simulink model "Modelo_R2023b"  (R2023b)
settings: Solver=VariableStepAuto  StartTime=0.0  StopTime=10.0  RelTol=1e-3
model workspace (MAT data in the model file):
  DC_Joint_J = 0.192319441127
  DC_Motor_D = 0.4
  DC_Motor_H = 0.192915716702
  DC_Motor_I = 1
  DC_Motor_J = 0.2131632295
  DC_Motor_Lower_Sat_Ref = -18
  DC_Motor_NLC = 0.11
  DC_Motor_NLS = 10000
  DC_Motor_P = 0.20625
  DC_Motor_ST = 0.0494309
  DC_Motor_TG = 0.95
  DC_Motor_Upper_Sat_Ref = 18
  DC_Motor_V = 12
  DRV_Deadzone_U = 128
  DRV_Motor_BTH = 0.001
  DRV_Motor_ETH = 0.15625
  DRV_Motor_FDR = 0.195188957589
  DRV_Motor_RTH = 0.001
  DRV_Motor_TBR = 0.10371374274
  MOTOR_Period_T = 0.01
  MOTOR_WHEEL_LPF : object (value not decoded)
  Robot_L = 0.15
  Robot_W = 0.15
  Robot_init_th = 0
  Robot_init_x = 0
  Robot_init_y = 0
  Robot_mm_to_m = 0.001
  Robot_wheel_radius = 0.05
  Robot_wheel_x_offset = 150
  Robot_wheel_y_offset = 102.5
  Robot_wheel_z_offset = 2
  Roller_Contact_df = 0.3
  Roller_Contact_dm = 1000
  Roller_Contact_sf = 0.5
  Roller_Contact_st = 1000000
  Roller_Joint_Friction = 0
  SIM_Base_Period_T = 0.001
  SIM_CTRL_Period_T = 0.1
  SIM_Floor_Height = 8.7
  SIM_Floor_Thick = 0.2
  SIM_Floor_Width = 9
  Sig : Simulink.Signal (value not decoded)
  Traj_ref = [0 0.1 0.2 0.3 0.4 0.5 0.6 0.7 0.8 0.9 1 0 ... (22 elements, 11x2)]
undefined symbols (not defined in the file): DiscIntNeverNeededParam, X, Y, Z
libraries: sm_lib x185, nesl_utility x37, fl_lib x32, ee_lib x12, simulink x8, aerolibconvert2 x4, cstblocks x4, sharedtransform x1, dspsigops x1
(part 4 of 4)

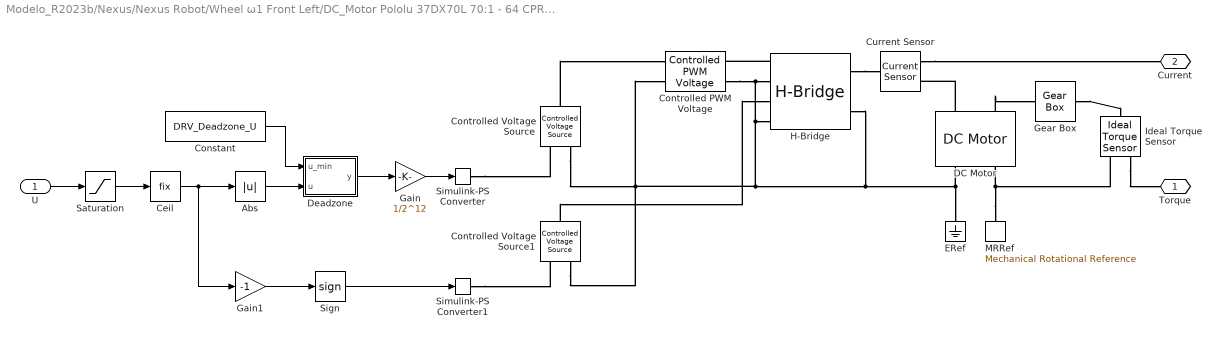
== system Modelo_R2023b/Nexus/Nexus Robot/Wheel ω1 Front Left/DC_Motor Pololu 37DX70L 70:1 - 64 CPR/Electrical ==
  U : Inport
  Abs : Abs  SaturateOnIntegerOverflow=off
  Ceil : Rounding  Operator=fix
  Constant : Constant  Value=DRV_Deadzone_U
  Controlled PWM Voltage : ee_lib/Integrated Circuits/Controlled PWM Voltage  F=1526 Hz  TD=0 s  pulse_width_offset=0 s  pulse_min=0 s  pwm_or_av=2  event_type=1  sample_time=5e-6 s  Vmin=0 V  Vmax=1 V  Vm=5 V  u_min=0  u_max=1
  Controlled Voltage Source : fl_lib/Electrical/Electrical Sources/Controlled Voltage Source
  Controlled Voltage Source1 : fl_lib/Electrical/Electrical Sources/Controlled Voltage Source
  Current Sensor : fl_lib/Electrical/Electrical Sensors/Current Sensor
  DC Motor : ee_lib/Electromechanical/Brushed Motors/DC Motor  field_option=ee.enum.field_option.pm  Rf=100 Ohm  Lf=1 H  Laf=0.15 H  If0=0 A  parameterization=ee.enum.dcparam_option.torque_speed  Ra=DC_Motor_R Ohm  La=DC_Motor_H H  emf_or_torque=ee.enum.emf_or_torque.kv  Kv=DC_Motor_K V/(rad/s)  Ki=6.876e-04 N*m/A  T_stall=DC_Motor_ST N*m  w_max=DC_Motor_NLS rpm  w_rated=150 rpm  P_rated=10 W  V_rated=nomV V  lam_param=ee.enum.lam_param.current  i_noload=0.11 A  V_i_noload=nomV V  J=DC_Motor_J kg*m^2  lam=DC_Motor_D N*m/(rad/s)  speed0=0 rpm  enable_fault_armature=simscape.enum.onoff.off  rev_faulted=1 / 3  G_faulted_armature=1e-5 S  fault_trigger_armature=ee.enum.faults.faultTrigger.temporal  t_fault_armature=1 s  max_permissible_current_armature=inf A  t_fail_on_current_armature=1 s  enable_fault_field=simscape.enum.onoff.off  G_faulted_field=1e-5 S  fault_trigger_field=ee.enum.faults.faultTrigger.temporal  t_fault_field=1 s  max_permissible_current_field=inf A  t_fail_on_current_field=1 s  fault_action=simscape.enum.assert.action.none  alpha=3.93e-3 1/K  Tmeas=25 degC  thermal_mass=100 J/K  initial_temperature=25 degC
  Deadzone : MATLAB Function  TreatAsAtomicUnit=on
  ERef : fl_lib/Electrical/Electrical Elements/Electrical Reference
  Gain : Gain  Gain=1/2^12
  Gain1 : Gain  Gain=-1
  Gear Box : fl_lib/Mechanical/Mechanisms/Gear Box  ratio=70  t_in_specify=off  t_in_priority=None  t_in=0 N*m  t_in_nominal_specify=off  t_in_nominal_unit=N*m  t_in_nominal_value=1  t_out_specify=off  t_out_priority=None  t_out=0 N*m  t_out_nominal_specify=off  t_out_nominal_unit=N*m  t_out_nominal_value=1
  H-Bridge : ee_lib/Semiconductors & Converters/Converters/H-Bridge  supply_ports=ee.enum.supply_ports.hidesupply  pwm_or_av=ee.enum.pwm_or_av.averaged  regenerative_braking_mode=ee.enum.converters.regenerative_braking_mode.always_enabled  discontinuous=ee.enum.current_profile.continuous  freewheeling_mode=ee.enum.converters.freewheeling_mode.one_switch_one_diode  Rload=3.38+0.1 Ohm  Lload=1e-5 H  F=4 kHz  Venable=DRV_Motor_ETH V  Vmax=5 V  Vreverse=DRV_Motor_RTH V  Vbrake=DRV_Motor_BTH V  Vm=nomV V  Ron=DRV_Motor_TBR Ohm  Don=DRV_Motor_FDR Ohm  Goff=1e-6 S  Tmeas=298.15 K  Ron2=0.1 Ohm  Don2=0.05 Ohm  Tmeas2=398.15 K  thermal_mass=100 J/K  initial_temperature=298.15 K
  Ideal Torque Sensor : fl_lib/Mechanical/Mechanical Sensors/Ideal Torque Sensor
  MRRef : fl_lib/Mechanical/Rotational Elements/Mechanical Rotational Reference
  Saturation : Saturate  UpperLimit=4096  LowerLimit=-4096
  Sign : Signum
  Simulink-PS Converter : nesl_utility/Simulink-PS Converter  PhysicalDomain=network_engine_domain  SubClassName=ps_input  LeftPortType=input  RightPortType=output  PseudoPeriodic=off  Frequencies=[]  NoiseDistribution=none  NoiseParameters=[]  Unit=V  AffineConversion=off  FilteringAndDerivatives=provide  SimscapeFilterOrder=1  InputFilterTimeConstant=0.001  UdotUserProvided=0
  Simulink-PS Converter1 : nesl_utility/Simulink-PS Converter  PhysicalDomain=network_engine_domain  SubClassName=ps_input  LeftPortType=input  RightPortType=output  PseudoPeriodic=off  Frequencies=[]  NoiseDistribution=none  NoiseParameters=[]  Unit=V  AffineConversion=off  FilteringAndDerivatives=provide  SimscapeFilterOrder=1  InputFilterTimeConstant=0.001  UdotUserProvided=0
  Torque : PMIOPort  Side=Right
  Current : PMIOPort  Port=2  Side=Right
  wires:
  Saturation/1 -> Ceil/1
  Sign/1 -> Simulink-PS Converter1/1
  Gain/1 -> Simulink-PS Converter/1
  U/1 -> Saturation/1
  Abs/1 -> Deadzone/2(u)
  Ceil/1 -> Gain1/1, Abs/1
  Deadzone/1(y) -> Gain/1
  Gain1/1 -> Sign/1
  Constant/1 -> Deadzone/1(u_min)
  connections:
  H-Bridge/RConn2 -- DC Motor/RConn1 -- ERef/LConn1 -- Controlled Voltage Source1/RConn2 -- Controlled Voltage Source/RConn2 -- Controlled PWM Voltage/LConn2 -- H-Bridge/LConn4 -- H-Bridge/LConn2 -- Controlled PWM Voltage/RConn2
  MRRef/LConn1 -- Ideal Torque Sensor/RConn1 -- DC Motor/RConn2
  H-Bridge/RConn1 -- Current Sensor/LConn1
  DC Motor/LConn1 -- Current Sensor/RConn2
  H-Bridge/LConn1 -- Controlled PWM Voltage/RConn1
  Current Sensor/RConn1 -- Current/RConn1
  Controlled Voltage Source/LConn1 -- Controlled PWM Voltage/LConn1
  Simulink-PS Converter/RConn1 -- Controlled Voltage Source/RConn1
  Ideal Torque Sensor/RConn2 -- Torque/RConn1
  DC Motor/LConn2 -- Gear Box/LConn1
  Gear Box/RConn1 -- Ideal Torque Sensor/LConn1
  Simulink-PS Converter1/RConn1 -- Controlled Voltage Source1/RConn1
  Controlled Voltage Source1/LConn1 -- H-Bridge/LConn3

== system Modelo_R2023b/Nexus/Nexus Robot/Wheel ω1 Front Left/DC_Motor Pololu 37DX70L 70:1 - 64 CPR/Mechanics ==
  Axis : sm_lib/Body Elements/File Solid  ExtGeomFileName=c_MG37D_Eje.stp  UnitType=FromFile  ExtGeomFileUnits=m  StepReaderType=HEX  ExportConvexHullGeometry=off  InertiaType=CalculateFromGeometry  Mass=1  MassUnits=kg  CenterOfMass=[0 0 0]  CenterOfMassUnits=m  MomentsOfInertia=[1 1 1]  MomentsOfInertiaUnits=kg*m^2  ProductsOfInertia=[0 0 0]  ProductsOfInertiaUnits=kg*m^2  BasedOnType=Density  Density=7850  DensityUnits=kg/m^3  DoExposeReferenceFrame=on  SerializedFrames=<Frames><Frame><Id>Frame1</Id><Value><Name>F1</Name><Origin><Source>GeometricFeature</Source><FeatureName>circular curve 6</FeatureName></Origin><PrimaryAxis><DefinedDirection>+Z</DefinedDirection><Source>ReferenceFrame</Source><SourceDirection>+Z</SourceDirection><FeatureName></FeatureName></PrimaryAxis><SecondaryAxis><DefinedDirection>+X</DefinedDirection><Source>ReferenceFrame</Source><SourceDirection>+X</SourceDirection><FeatureName></FeatureName></SecondaryAxis></Value></Frame></Frames>  GraphicType=FromGeometry  MarkerShape=Sphere  MarkerSize=10  GraphicVisPropType=SimpleVisualProperties  GraphicDiffuseColor=[0.8 0.8 0.8]  GraphicSpecularColor=[0.5 0.5 0.5 1.0]  GraphicAmbientColor=[0.15 0.15 0.15 1.0]  GraphicEmissiveColor=[0.0 0.0 0.0 1.0]  GraphicShininess=75  GraphicOpacity=1.0
  PS Gain : fl_lib/Physical Signals/Functions/PS Gain  gain=DC_Motor_TG
  Revolute Joint : sm_lib/Joints/Revolute Joint  JointMode=Normal  SenseConstraintForce=off  SenseConstraintForceX=off  SenseConstraintForceY=off  SenseConstraintForceZ=off  SenseConstraintTorque=off  SenseConstraintTorqueX=off  SenseConstraintTorqueY=off  SenseConstraintTorqueZ=off  SenseTotalForce=off  SenseTotalForceX=off  SenseTotalForceY=off  SenseTotalForceZ=off  SenseTotalTorque=off  SenseTotalTorqueX=off  SenseTotalTorqueY=off  SenseTotalTorqueZ=off  CompositeWrenchDir=FollowerOnBase  CompositeWrenchFrame=BaseFrame  EquilibriumPosition=0  EquilibriumPositionUnits=deg  SpringStiffness=0  SpringStiffnessUnits=N*m/deg  DampingCoefficient=DC_Joint_J  DampingCoefficientUnits=N*m/(rad/s)  TorqueActuationMode=InputTorque  MotionActuationMode=ComputedMotion  SensePosition=on  SenseVelocity=on  SenseAcceleration=off  SenseTorqueForce=off  SenseLowerLimitTorqueForce=off  SenseUpperLimitTorqueForce=off  LowerLimitSpecify=off  LowerLimitBound=-90  LowerLimitBoundUnits=deg  LowerLimitStiffness=1e4  LowerLimitStiffnessUnits=N*m/deg  LowerLimitDamping=10  LowerLimitDampingUnits=N*m/(deg/s)  LowerLimitTransitionRegionWidth=0.1  LowerLimitTransitionRegionWidthUnits=deg  UpperLimitSpecify=off  UpperLimitBound=90  UpperLimitBoundUnits=deg  UpperLimitStiffness=1e4  UpperLimitStiffnessUnits=N*m/deg  UpperLimitDamping=10  UpperLimitDampingUnits=N*m/(deg/s)  UpperLimitTransitionRegionWidth=0.1  UpperLimitTransitionRegionWidthUnits=deg  PositionTargetSpecify=off  PositionTargetPriority=High  PositionTargetValue=0  PositionTargetValueUnits=deg  VelocityTargetSpecify=off  VelocityTargetPriority=High  VelocityTargetValue=0  VelocityTargetValueUnits=deg/s
  FW : PMIOPort  Side=Left
  τ : PMIOPort  Port=2  Side=Left
  Wheel : PMIOPort  Port=3  Side=Right
  θ : PMIOPort  Port=4  Side=Right
  ω : PMIOPort  Port=5  Side=Right
  connections:
  Revolute Joint/RConn2 -- θ/RConn1
  FW/RConn1 -- Revolute Joint/LConn1
  Axis/RConn1 -- Revolute Joint/RConn1
  PS Gain/LConn1 -- τ/RConn1
  Revolute Joint/RConn3 -- ω/RConn1
  Revolute Joint/LConn2 -- PS Gain/RConn1
  Wheel/RConn1 -- Axis/LConn1

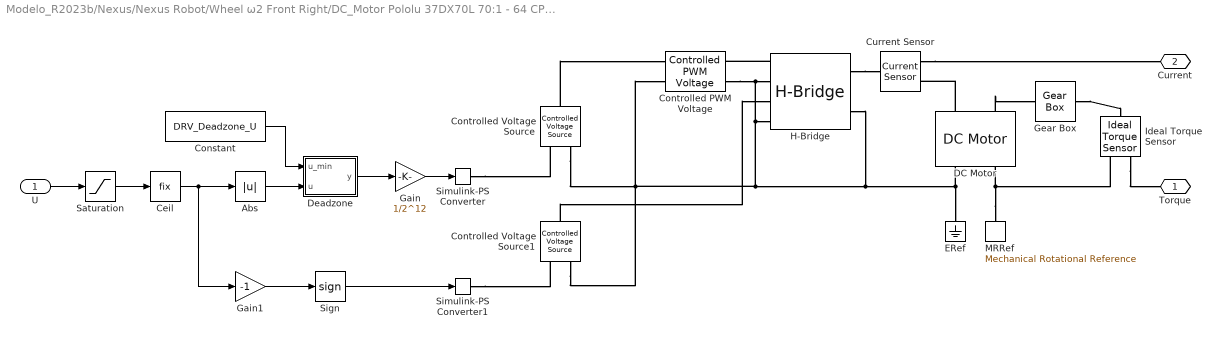
== system Modelo_R2023b/Nexus/Nexus Robot/Wheel ω2 Front Right/DC_Motor Pololu 37DX70L 70:1 - 64 CPR/Electrical ==
  U : Inport
  Abs : Abs  SaturateOnIntegerOverflow=off
  Ceil : Rounding  Operator=fix
  Constant : Constant  Value=DRV_Deadzone_U
  Controlled PWM Voltage : ee_lib/Integrated Circuits/Controlled PWM Voltage  F=1526 Hz  TD=0 s  pulse_width_offset=0 s  pulse_min=0 s  pwm_or_av=2  event_type=1  sample_time=5e-6 s  Vmin=0 V  Vmax=1 V  Vm=5 V  u_min=0  u_max=1
  Controlled Voltage Source : fl_lib/Electrical/Electrical Sources/Controlled Voltage Source
  Controlled Voltage Source1 : fl_lib/Electrical/Electrical Sources/Controlled Voltage Source
  Current Sensor : fl_lib/Electrical/Electrical Sensors/Current Sensor
  DC Motor : ee_lib/Electromechanical/Brushed Motors/DC Motor  field_option=ee.enum.field_option.pm  Rf=100 Ohm  Lf=1 H  Laf=0.15 H  If0=0 A  parameterization=ee.enum.dcparam_option.torque_speed  Ra=DC_Motor_R Ohm  La=DC_Motor_H H  emf_or_torque=ee.enum.emf_or_torque.kv  Kv=DC_Motor_K V/(rad/s)  Ki=6.876e-04 N*m/A  T_stall=DC_Motor_ST N*m  w_max=DC_Motor_NLS rpm  w_rated=150 rpm  P_rated=10 W  V_rated=nomV V  lam_param=ee.enum.lam_param.current  i_noload=0.11 A  V_i_noload=nomV V  J=DC_Motor_J kg*m^2  lam=DC_Motor_D N*m/(rad/s)  speed0=0 rpm  enable_fault_armature=simscape.enum.onoff.off  rev_faulted=1 / 3  G_faulted_armature=1e-5 S  fault_trigger_armature=ee.enum.faults.faultTrigger.temporal  t_fault_armature=1 s  max_permissible_current_armature=inf A  t_fail_on_current_armature=1 s  enable_fault_field=simscape.enum.onoff.off  G_faulted_field=1e-5 S  fault_trigger_field=ee.enum.faults.faultTrigger.temporal  t_fault_field=1 s  max_permissible_current_field=inf A  t_fail_on_current_field=1 s  fault_action=simscape.enum.assert.action.none  alpha=3.93e-3 1/K  Tmeas=25 degC  thermal_mass=100 J/K  initial_temperature=25 degC
  Deadzone : MATLAB Function  TreatAsAtomicUnit=on
  ERef : fl_lib/Electrical/Electrical Elements/Electrical Reference
  Gain : Gain  Gain=1/2^12
  Gain1 : Gain  Gain=-1
  Gear Box : fl_lib/Mechanical/Mechanisms/Gear Box  ratio=70  t_in_specify=off  t_in_priority=None  t_in=0 N*m  t_in_nominal_specify=off  t_in_nominal_unit=N*m  t_in_nominal_value=1  t_out_specify=off  t_out_priority=None  t_out=0 N*m  t_out_nominal_specify=off  t_out_nominal_unit=N*m  t_out_nominal_value=1
  H-Bridge : ee_lib/Semiconductors & Converters/Converters/H-Bridge  supply_ports=ee.enum.supply_ports.hidesupply  pwm_or_av=ee.enum.pwm_or_av.averaged  regenerative_braking_mode=ee.enum.converters.regenerative_braking_mode.always_enabled  discontinuous=ee.enum.current_profile.continuous  freewheeling_mode=ee.enum.converters.freewheeling_mode.one_switch_one_diode  Rload=3.38+0.1 Ohm  Lload=1e-5 H  F=4 kHz  Venable=DRV_Motor_ETH V  Vmax=5 V  Vreverse=DRV_Motor_RTH V  Vbrake=DRV_Motor_BTH V  Vm=nomV V  Ron=DRV_Motor_TBR Ohm  Don=DRV_Motor_FDR Ohm  Goff=1e-6 S  Tmeas=298.15 K  Ron2=0.1 Ohm  Don2=0.05 Ohm  Tmeas2=398.15 K  thermal_mass=100 J/K  initial_temperature=298.15 K
  Ideal Torque Sensor : fl_lib/Mechanical/Mechanical Sensors/Ideal Torque Sensor
  MRRef : fl_lib/Mechanical/Rotational Elements/Mechanical Rotational Reference
  Saturation : Saturate  UpperLimit=4096  LowerLimit=-4096
  Sign : Signum
  Simulink-PS Converter : nesl_utility/Simulink-PS Converter  PhysicalDomain=network_engine_domain  SubClassName=ps_input  LeftPortType=input  RightPortType=output  PseudoPeriodic=off  Frequencies=[]  NoiseDistribution=none  NoiseParameters=[]  Unit=V  AffineConversion=off  FilteringAndDerivatives=provide  SimscapeFilterOrder=1  InputFilterTimeConstant=0.001  UdotUserProvided=0
  Simulink-PS Converter1 : nesl_utility/Simulink-PS Converter  PhysicalDomain=network_engine_domain  SubClassName=ps_input  LeftPortType=input  RightPortType=output  PseudoPeriodic=off  Frequencies=[]  NoiseDistribution=none  NoiseParameters=[]  Unit=V  AffineConversion=off  FilteringAndDerivatives=provide  SimscapeFilterOrder=1  InputFilterTimeConstant=0.001  UdotUserProvided=0
  Torque : PMIOPort  Side=Right
  Current : PMIOPort  Port=2  Side=Right
  wires:
  Saturation/1 -> Ceil/1
  Sign/1 -> Simulink-PS Converter1/1
  Gain/1 -> Simulink-PS Converter/1
  U/1 -> Saturation/1
  Abs/1 -> Deadzone/2(u)
  Ceil/1 -> Gain1/1, Abs/1
  Deadzone/1(y) -> Gain/1
  Gain1/1 -> Sign/1
  Constant/1 -> Deadzone/1(u_min)
  connections:
  H-Bridge/RConn2 -- DC Motor/RConn1 -- ERef/LConn1 -- Controlled Voltage Source1/RConn2 -- Controlled Voltage Source/RConn2 -- Controlled PWM Voltage/LConn2 -- H-Bridge/LConn4 -- H-Bridge/LConn2 -- Controlled PWM Voltage/RConn2
  MRRef/LConn1 -- Ideal Torque Sensor/RConn1 -- DC Motor/RConn2
  H-Bridge/RConn1 -- Current Sensor/LConn1
  DC Motor/LConn1 -- Current Sensor/RConn2
  H-Bridge/LConn1 -- Controlled PWM Voltage/RConn1
  Current Sensor/RConn1 -- Current/RConn1
  Controlled Voltage Source/LConn1 -- Controlled PWM Voltage/LConn1
  Simulink-PS Converter/RConn1 -- Controlled Voltage Source/RConn1
  Ideal Torque Sensor/RConn2 -- Torque/RConn1
  DC Motor/LConn2 -- Gear Box/LConn1
  Gear Box/RConn1 -- Ideal Torque Sensor/LConn1
  Simulink-PS Converter1/RConn1 -- Controlled Voltage Source1/RConn1
  Controlled Voltage Source1/LConn1 -- H-Bridge/LConn3

== system Modelo_R2023b/Nexus/Nexus Robot/Wheel ω2 Front Right/DC_Motor Pololu 37DX70L 70:1 - 64 CPR/Mechanics ==
  Axis : sm_lib/Body Elements/File Solid  ExtGeomFileName=c_MG37D_Eje.stp  UnitType=FromFile  ExtGeomFileUnits=m  StepReaderType=HEX  ExportConvexHullGeometry=off  InertiaType=CalculateFromGeometry  Mass=1  MassUnits=kg  CenterOfMass=[0 0 0]  CenterOfMassUnits=m  MomentsOfInertia=[1 1 1]  MomentsOfInertiaUnits=kg*m^2  ProductsOfInertia=[0 0 0]  ProductsOfInertiaUnits=kg*m^2  BasedOnType=Density  Density=7850  DensityUnits=kg/m^3  DoExposeReferenceFrame=on  SerializedFrames=<Frames><Frame><Id>Frame1</Id><Value><Name>F1</Name><Origin><Source>GeometricFeature</Source><FeatureName>circular curve 6</FeatureName></Origin><PrimaryAxis><DefinedDirection>+Z</DefinedDirection><Source>ReferenceFrame</Source><SourceDirection>+Z</SourceDirection><FeatureName></FeatureName></PrimaryAxis><SecondaryAxis><DefinedDirection>+X</DefinedDirection><Source>ReferenceFrame</Source><SourceDirection>+X</SourceDirection><FeatureName></FeatureName></SecondaryAxis></Value></Frame></Frames>  GraphicType=FromGeometry  MarkerShape=Sphere  MarkerSize=10  GraphicVisPropType=SimpleVisualProperties  GraphicDiffuseColor=[0.8 0.8 0.8]  GraphicSpecularColor=[0.5 0.5 0.5 1.0]  GraphicAmbientColor=[0.15 0.15 0.15 1.0]  GraphicEmissiveColor=[0.0 0.0 0.0 1.0]  GraphicShininess=75  GraphicOpacity=1.0
  PS Gain : fl_lib/Physical Signals/Functions/PS Gain  gain=DC_Motor_TG
  Revolute Joint : sm_lib/Joints/Revolute Joint  JointMode=Normal  SenseConstraintForce=off  SenseConstraintForceX=off  SenseConstraintForceY=off  SenseConstraintForceZ=off  SenseConstraintTorque=off  SenseConstraintTorqueX=off  SenseConstraintTorqueY=off  SenseConstraintTorqueZ=off  SenseTotalForce=off  SenseTotalForceX=off  SenseTotalForceY=off  SenseTotalForceZ=off  SenseTotalTorque=off  SenseTotalTorqueX=off  SenseTotalTorqueY=off  SenseTotalTorqueZ=off  CompositeWrenchDir=FollowerOnBase  CompositeWrenchFrame=BaseFrame  EquilibriumPosition=0  EquilibriumPositionUnits=deg  SpringStiffness=0  SpringStiffnessUnits=N*m/deg  DampingCoefficient=DC_Joint_J  DampingCoefficientUnits=N*m/(rad/s)  TorqueActuationMode=InputTorque  MotionActuationMode=ComputedMotion  SensePosition=on  SenseVelocity=on  SenseAcceleration=off  SenseTorqueForce=off  SenseLowerLimitTorqueForce=off  SenseUpperLimitTorqueForce=off  LowerLimitSpecify=off  LowerLimitBound=-90  LowerLimitBoundUnits=deg  LowerLimitStiffness=1e4  LowerLimitStiffnessUnits=N*m/deg  LowerLimitDamping=10  LowerLimitDampingUnits=N*m/(deg/s)  LowerLimitTransitionRegionWidth=0.1  LowerLimitTransitionRegionWidthUnits=deg  UpperLimitSpecify=off  UpperLimitBound=90  UpperLimitBoundUnits=deg  UpperLimitStiffness=1e4  UpperLimitStiffnessUnits=N*m/deg  UpperLimitDamping=10  UpperLimitDampingUnits=N*m/(deg/s)  UpperLimitTransitionRegionWidth=0.1  UpperLimitTransitionRegionWidthUnits=deg  PositionTargetSpecify=off  PositionTargetPriority=High  PositionTargetValue=0  PositionTargetValueUnits=deg  VelocityTargetSpecify=off  VelocityTargetPriority=High  VelocityTargetValue=0  VelocityTargetValueUnits=deg/s
  FW : PMIOPort  Side=Left
  τ : PMIOPort  Port=2  Side=Left
  Wheel : PMIOPort  Port=3  Side=Right
  θ : PMIOPort  Port=4  Side=Right
  ω : PMIOPort  Port=5  Side=Right
  connections:
  Revolute Joint/RConn2 -- θ/RConn1
  FW/RConn1 -- Revolute Joint/LConn1
  Axis/RConn1 -- Revolute Joint/RConn1
  PS Gain/LConn1 -- τ/RConn1
  Revolute Joint/RConn3 -- ω/RConn1
  Revolute Joint/LConn2 -- PS Gain/RConn1
  Wheel/RConn1 -- Axis/LConn1

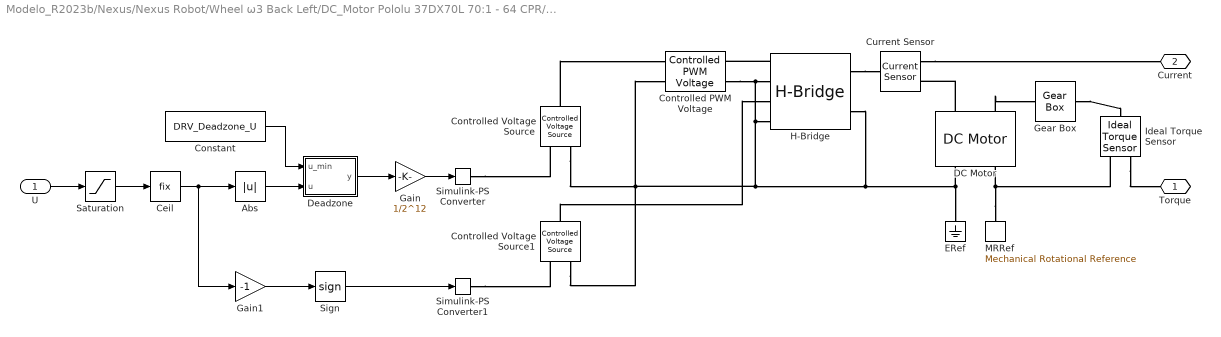
== system Modelo_R2023b/Nexus/Nexus Robot/Wheel ω3 Back Left/DC_Motor Pololu 37DX70L 70:1 - 64 CPR/Electrical ==
  U : Inport
  Abs : Abs  SaturateOnIntegerOverflow=off
  Ceil : Rounding  Operator=fix
  Constant : Constant  Value=DRV_Deadzone_U
  Controlled PWM Voltage : ee_lib/Integrated Circuits/Controlled PWM Voltage  F=1526 Hz  TD=0 s  pulse_width_offset=0 s  pulse_min=0 s  pwm_or_av=2  event_type=1  sample_time=5e-6 s  Vmin=0 V  Vmax=1 V  Vm=5 V  u_min=0  u_max=1
  Controlled Voltage Source : fl_lib/Electrical/Electrical Sources/Controlled Voltage Source
  Controlled Voltage Source1 : fl_lib/Electrical/Electrical Sources/Controlled Voltage Source
  Current Sensor : fl_lib/Electrical/Electrical Sensors/Current Sensor
  DC Motor : ee_lib/Electromechanical/Brushed Motors/DC Motor  field_option=ee.enum.field_option.pm  Rf=100 Ohm  Lf=1 H  Laf=0.15 H  If0=0 A  parameterization=ee.enum.dcparam_option.torque_speed  Ra=DC_Motor_R Ohm  La=DC_Motor_H H  emf_or_torque=ee.enum.emf_or_torque.kv  Kv=DC_Motor_K V/(rad/s)  Ki=6.876e-04 N*m/A  T_stall=DC_Motor_ST N*m  w_max=DC_Motor_NLS rpm  w_rated=150 rpm  P_rated=10 W  V_rated=nomV V  lam_param=ee.enum.lam_param.current  i_noload=0.11 A  V_i_noload=nomV V  J=DC_Motor_J kg*m^2  lam=DC_Motor_D N*m/(rad/s)  speed0=0 rpm  enable_fault_armature=simscape.enum.onoff.off  rev_faulted=1 / 3  G_faulted_armature=1e-5 S  fault_trigger_armature=ee.enum.faults.faultTrigger.temporal  t_fault_armature=1 s  max_permissible_current_armature=inf A  t_fail_on_current_armature=1 s  enable_fault_field=simscape.enum.onoff.off  G_faulted_field=1e-5 S  fault_trigger_field=ee.enum.faults.faultTrigger.temporal  t_fault_field=1 s  max_permissible_current_field=inf A  t_fail_on_current_field=1 s  fault_action=simscape.enum.assert.action.none  alpha=3.93e-3 1/K  Tmeas=25 degC  thermal_mass=100 J/K  initial_temperature=25 degC
  Deadzone : MATLAB Function  TreatAsAtomicUnit=on
  ERef : fl_lib/Electrical/Electrical Elements/Electrical Reference
  Gain : Gain  Gain=1/2^12
  Gain1 : Gain  Gain=-1
  Gear Box : fl_lib/Mechanical/Mechanisms/Gear Box  ratio=70  t_in_specify=off  t_in_priority=None  t_in=0 N*m  t_in_nominal_specify=off  t_in_nominal_unit=N*m  t_in_nominal_value=1  t_out_specify=off  t_out_priority=None  t_out=0 N*m  t_out_nominal_specify=off  t_out_nominal_unit=N*m  t_out_nominal_value=1
  H-Bridge : ee_lib/Semiconductors & Converters/Converters/H-Bridge  supply_ports=ee.enum.supply_ports.hidesupply  pwm_or_av=ee.enum.pwm_or_av.averaged  regenerative_braking_mode=ee.enum.converters.regenerative_braking_mode.always_enabled  discontinuous=ee.enum.current_profile.continuous  freewheeling_mode=ee.enum.converters.freewheeling_mode.one_switch_one_diode  Rload=3.38+0.1 Ohm  Lload=1e-5 H  F=4 kHz  Venable=DRV_Motor_ETH V  Vmax=5 V  Vreverse=DRV_Motor_RTH V  Vbrake=DRV_Motor_BTH V  Vm=nomV V  Ron=DRV_Motor_TBR Ohm  Don=DRV_Motor_FDR Ohm  Goff=1e-6 S  Tmeas=298.15 K  Ron2=0.1 Ohm  Don2=0.05 Ohm  Tmeas2=398.15 K  thermal_mass=100 J/K  initial_temperature=298.15 K
  Ideal Torque Sensor : fl_lib/Mechanical/Mechanical Sensors/Ideal Torque Sensor
  MRRef : fl_lib/Mechanical/Rotational Elements/Mechanical Rotational Reference
  Saturation : Saturate  UpperLimit=4096  LowerLimit=-4096
  Sign : Signum
  Simulink-PS Converter : nesl_utility/Simulink-PS Converter  PhysicalDomain=network_engine_domain  SubClassName=ps_input  LeftPortType=input  RightPortType=output  PseudoPeriodic=off  Frequencies=[]  NoiseDistribution=none  NoiseParameters=[]  Unit=V  AffineConversion=off  FilteringAndDerivatives=provide  SimscapeFilterOrder=1  InputFilterTimeConstant=0.001  UdotUserProvided=0
  Simulink-PS Converter1 : nesl_utility/Simulink-PS Converter  PhysicalDomain=network_engine_domain  SubClassName=ps_input  LeftPortType=input  RightPortType=output  PseudoPeriodic=off  Frequencies=[]  NoiseDistribution=none  NoiseParameters=[]  Unit=V  AffineConversion=off  FilteringAndDerivatives=provide  SimscapeFilterOrder=1  InputFilterTimeConstant=0.001  UdotUserProvided=0
  Torque : PMIOPort  Side=Right
  Current : PMIOPort  Port=2  Side=Right
  wires:
  Saturation/1 -> Ceil/1
  Sign/1 -> Simulink-PS Converter1/1
  Gain/1 -> Simulink-PS Converter/1
  U/1 -> Saturation/1
  Abs/1 -> Deadzone/2(u)
  Ceil/1 -> Gain1/1, Abs/1
  Deadzone/1(y) -> Gain/1
  Gain1/1 -> Sign/1
  Constant/1 -> Deadzone/1(u_min)
  connections:
  H-Bridge/RConn2 -- DC Motor/RConn1 -- ERef/LConn1 -- Controlled Voltage Source1/RConn2 -- Controlled Voltage Source/RConn2 -- Controlled PWM Voltage/LConn2 -- H-Bridge/LConn4 -- H-Bridge/LConn2 -- Controlled PWM Voltage/RConn2
  MRRef/LConn1 -- Ideal Torque Sensor/RConn1 -- DC Motor/RConn2
  H-Bridge/RConn1 -- Current Sensor/LConn1
  DC Motor/LConn1 -- Current Sensor/RConn2
  H-Bridge/LConn1 -- Controlled PWM Voltage/RConn1
  Current Sensor/RConn1 -- Current/RConn1
  Controlled Voltage Source/LConn1 -- Controlled PWM Voltage/LConn1
  Simulink-PS Converter/RConn1 -- Controlled Voltage Source/RConn1
  Ideal Torque Sensor/RConn2 -- Torque/RConn1
  DC Motor/LConn2 -- Gear Box/LConn1
  Gear Box/RConn1 -- Ideal Torque Sensor/LConn1
  Simulink-PS Converter1/RConn1 -- Controlled Voltage Source1/RConn1
  Controlled Voltage Source1/LConn1 -- H-Bridge/LConn3

== system Modelo_R2023b/Nexus/Nexus Robot/Wheel ω3 Back Left/DC_Motor Pololu 37DX70L 70:1 - 64 CPR/Mechanics ==
  Axis : sm_lib/Body Elements/File Solid  ExtGeomFileName=c_MG37D_Eje.stp  UnitType=FromFile  ExtGeomFileUnits=m  StepReaderType=HEX  ExportConvexHullGeometry=off  InertiaType=CalculateFromGeometry  Mass=1  MassUnits=kg  CenterOfMass=[0 0 0]  CenterOfMassUnits=m  MomentsOfInertia=[1 1 1]  MomentsOfInertiaUnits=kg*m^2  ProductsOfInertia=[0 0 0]  ProductsOfInertiaUnits=kg*m^2  BasedOnType=Density  Density=7850  DensityUnits=kg/m^3  DoExposeReferenceFrame=on  SerializedFrames=<Frames><Frame><Id>Frame1</Id><Value><Name>F1</Name><Origin><Source>GeometricFeature</Source><FeatureName>circular curve 6</FeatureName></Origin><PrimaryAxis><DefinedDirection>+Z</DefinedDirection><Source>ReferenceFrame</Source><SourceDirection>+Z</SourceDirection><FeatureName></FeatureName></PrimaryAxis><SecondaryAxis><DefinedDirection>+X</DefinedDirection><Source>ReferenceFrame</Source><SourceDirection>+X</SourceDirection><FeatureName></FeatureName></SecondaryAxis></Value></Frame></Frames>  GraphicType=FromGeometry  MarkerShape=Sphere  MarkerSize=10  GraphicVisPropType=SimpleVisualProperties  GraphicDiffuseColor=[0.8 0.8 0.8]  GraphicSpecularColor=[0.5 0.5 0.5 1.0]  GraphicAmbientColor=[0.15 0.15 0.15 1.0]  GraphicEmissiveColor=[0.0 0.0 0.0 1.0]  GraphicShininess=75  GraphicOpacity=1.0
  PS Gain : fl_lib/Physical Signals/Functions/PS Gain  gain=DC_Motor_TG
  Revolute Joint : sm_lib/Joints/Revolute Joint  JointMode=Normal  SenseConstraintForce=off  SenseConstraintForceX=off  SenseConstraintForceY=off  SenseConstraintForceZ=off  SenseConstraintTorque=off  SenseConstraintTorqueX=off  SenseConstraintTorqueY=off  SenseConstraintTorqueZ=off  SenseTotalForce=off  SenseTotalForceX=off  SenseTotalForceY=off  SenseTotalForceZ=off  SenseTotalTorque=off  SenseTotalTorqueX=off  SenseTotalTorqueY=off  SenseTotalTorqueZ=off  CompositeWrenchDir=FollowerOnBase  CompositeWrenchFrame=BaseFrame  EquilibriumPosition=0  EquilibriumPositionUnits=deg  SpringStiffness=0  SpringStiffnessUnits=N*m/deg  DampingCoefficient=DC_Joint_J  DampingCoefficientUnits=N*m/(rad/s)  TorqueActuationMode=InputTorque  MotionActuationMode=ComputedMotion  SensePosition=on  SenseVelocity=on  SenseAcceleration=off  SenseTorqueForce=off  SenseLowerLimitTorqueForce=off  SenseUpperLimitTorqueForce=off  LowerLimitSpecify=off  LowerLimitBound=-90  LowerLimitBoundUnits=deg  LowerLimitStiffness=1e4  LowerLimitStiffnessUnits=N*m/deg  LowerLimitDamping=10  LowerLimitDampingUnits=N*m/(deg/s)  LowerLimitTransitionRegionWidth=0.1  LowerLimitTransitionRegionWidthUnits=deg  UpperLimitSpecify=off  UpperLimitBound=90  UpperLimitBoundUnits=deg  UpperLimitStiffness=1e4  UpperLimitStiffnessUnits=N*m/deg  UpperLimitDamping=10  UpperLimitDampingUnits=N*m/(deg/s)  UpperLimitTransitionRegionWidth=0.1  UpperLimitTransitionRegionWidthUnits=deg  PositionTargetSpecify=off  PositionTargetPriority=High  PositionTargetValue=0  PositionTargetValueUnits=deg  VelocityTargetSpecify=off  VelocityTargetPriority=High  VelocityTargetValue=0  VelocityTargetValueUnits=deg/s
  FW : PMIOPort  Side=Left
  τ : PMIOPort  Port=2  Side=Left
  Wheel : PMIOPort  Port=3  Side=Right
  θ : PMIOPort  Port=4  Side=Right
  ω : PMIOPort  Port=5  Side=Right
  connections:
  Revolute Joint/RConn2 -- θ/RConn1
  FW/RConn1 -- Revolute Joint/LConn1
  Axis/RConn1 -- Revolute Joint/RConn1
  PS Gain/LConn1 -- τ/RConn1
  Revolute Joint/RConn3 -- ω/RConn1
  Revolute Joint/LConn2 -- PS Gain/RConn1
  Wheel/RConn1 -- Axis/LConn1

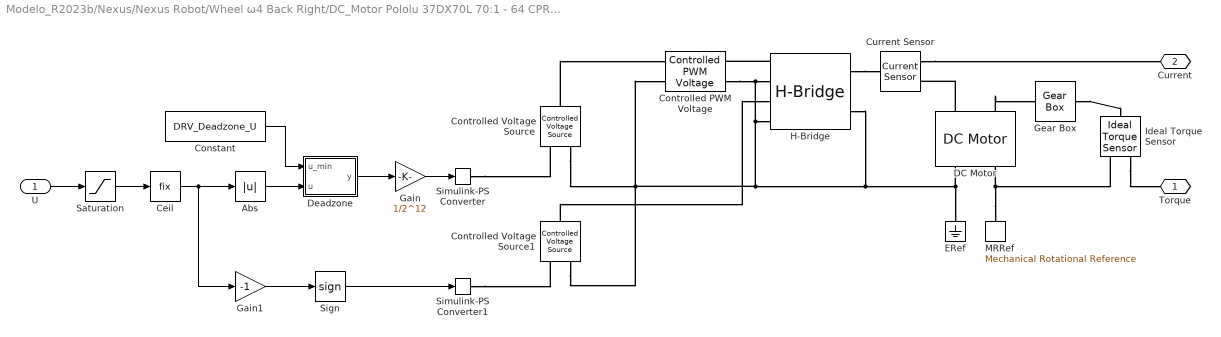
== system Modelo_R2023b/Nexus/Nexus Robot/Wheel ω4 Back Right/DC_Motor Pololu 37DX70L 70:1 - 64 CPR/Electrical ==
  U : Inport
  Abs : Abs  SaturateOnIntegerOverflow=off
  Ceil : Rounding  Operator=fix
  Constant : Constant  Value=DRV_Deadzone_U
  Controlled PWM Voltage : ee_lib/Integrated Circuits/Controlled PWM Voltage  F=1526 Hz  TD=0 s  pulse_width_offset=0 s  pulse_min=0 s  pwm_or_av=2  event_type=1  sample_time=5e-6 s  Vmin=0 V  Vmax=1 V  Vm=5 V  u_min=0  u_max=1
  Controlled Voltage Source : fl_lib/Electrical/Electrical Sources/Controlled Voltage Source
  Controlled Voltage Source1 : fl_lib/Electrical/Electrical Sources/Controlled Voltage Source
  Current Sensor : fl_lib/Electrical/Electrical Sensors/Current Sensor
  DC Motor : ee_lib/Electromechanical/Brushed Motors/DC Motor  field_option=ee.enum.field_option.pm  Rf=100 Ohm  Lf=1 H  Laf=0.15 H  If0=0 A  parameterization=ee.enum.dcparam_option.torque_speed  Ra=DC_Motor_R Ohm  La=DC_Motor_H H  emf_or_torque=ee.enum.emf_or_torque.kv  Kv=DC_Motor_K V/(rad/s)  Ki=6.876e-04 N*m/A  T_stall=DC_Motor_ST N*m  w_max=DC_Motor_NLS rpm  w_rated=150 rpm  P_rated=10 W  V_rated=nomV V  lam_param=ee.enum.lam_param.current  i_noload=0.11 A  V_i_noload=nomV V  J=DC_Motor_J kg*m^2  lam=DC_Motor_D N*m/(rad/s)  speed0=0 rpm  enable_fault_armature=simscape.enum.onoff.off  rev_faulted=1 / 3  G_faulted_armature=1e-5 S  fault_trigger_armature=ee.enum.faults.faultTrigger.temporal  t_fault_armature=1 s  max_permissible_current_armature=inf A  t_fail_on_current_armature=1 s  enable_fault_field=simscape.enum.onoff.off  G_faulted_field=1e-5 S  fault_trigger_field=ee.enum.faults.faultTrigger.temporal  t_fault_field=1 s  max_permissible_current_field=inf A  t_fail_on_current_field=1 s  fault_action=simscape.enum.assert.action.none  alpha=3.93e-3 1/K  Tmeas=25 degC  thermal_mass=100 J/K  initial_temperature=25 degC
  Deadzone : MATLAB Function  TreatAsAtomicUnit=on
  ERef : fl_lib/Electrical/Electrical Elements/Electrical Reference
  Gain : Gain  Gain=1/2^12
  Gain1 : Gain  Gain=-1
  Gear Box : fl_lib/Mechanical/Mechanisms/Gear Box  ratio=70  t_in_specify=off  t_in_priority=None  t_in=0 N*m  t_in_nominal_specify=off  t_in_nominal_unit=N*m  t_in_nominal_value=1  t_out_specify=off  t_out_priority=None  t_out=0 N*m  t_out_nominal_specify=off  t_out_nominal_unit=N*m  t_out_nominal_value=1
  H-Bridge : ee_lib/Semiconductors & Converters/Converters/H-Bridge  supply_ports=ee.enum.supply_ports.hidesupply  pwm_or_av=ee.enum.pwm_or_av.averaged  regenerative_braking_mode=ee.enum.converters.regenerative_braking_mode.always_enabled  discontinuous=ee.enum.current_profile.continuous  freewheeling_mode=ee.enum.converters.freewheeling_mode.one_switch_one_diode  Rload=3.38+0.1 Ohm  Lload=1e-5 H  F=4 kHz  Venable=DRV_Motor_ETH V  Vmax=5 V  Vreverse=DRV_Motor_RTH V  Vbrake=DRV_Motor_BTH V  Vm=nomV V  Ron=DRV_Motor_TBR Ohm  Don=DRV_Motor_FDR Ohm  Goff=1e-6 S  Tmeas=298.15 K  Ron2=0.1 Ohm  Don2=0.05 Ohm  Tmeas2=398.15 K  thermal_mass=100 J/K  initial_temperature=298.15 K
  Ideal Torque Sensor : fl_lib/Mechanical/Mechanical Sensors/Ideal Torque Sensor
  MRRef : fl_lib/Mechanical/Rotational Elements/Mechanical Rotational Reference
  Saturation : Saturate  UpperLimit=4096  LowerLimit=-4096
  Sign : Signum
  Simulink-PS Converter : nesl_utility/Simulink-PS Converter  PhysicalDomain=network_engine_domain  SubClassName=ps_input  LeftPortType=input  RightPortType=output  PseudoPeriodic=off  Frequencies=[]  NoiseDistribution=none  NoiseParameters=[]  Unit=V  AffineConversion=off  FilteringAndDerivatives=provide  SimscapeFilterOrder=1  InputFilterTimeConstant=0.001  UdotUserProvided=0
  Simulink-PS Converter1 : nesl_utility/Simulink-PS Converter  PhysicalDomain=network_engine_domain  SubClassName=ps_input  LeftPortType=input  RightPortType=output  PseudoPeriodic=off  Frequencies=[]  NoiseDistribution=none  NoiseParameters=[]  Unit=V  AffineConversion=off  FilteringAndDerivatives=provide  SimscapeFilterOrder=1  InputFilterTimeConstant=0.001  UdotUserProvided=0
  Torque : PMIOPort  Side=Right
  Current : PMIOPort  Port=2  Side=Right
  wires:
  Saturation/1 -> Ceil/1
  Sign/1 -> Simulink-PS Converter1/1
  Gain/1 -> Simulink-PS Converter/1
  U/1 -> Saturation/1
  Abs/1 -> Deadzone/2(u)
  Ceil/1 -> Gain1/1, Abs/1
  Deadzone/1(y) -> Gain/1
  Gain1/1 -> Sign/1
  Constant/1 -> Deadzone/1(u_min)
  connections:
  H-Bridge/RConn2 -- DC Motor/RConn1 -- ERef/LConn1 -- Controlled Voltage Source1/RConn2 -- Controlled Voltage Source/RConn2 -- Controlled PWM Voltage/LConn2 -- H-Bridge/LConn4 -- H-Bridge/LConn2 -- Controlled PWM Voltage/RConn2
  MRRef/LConn1 -- Ideal Torque Sensor/RConn1 -- DC Motor/RConn2
  H-Bridge/RConn1 -- Current Sensor/LConn1
  DC Motor/LConn1 -- Current Sensor/RConn2
  H-Bridge/LConn1 -- Controlled PWM Voltage/RConn1
  Current Sensor/RConn1 -- Current/RConn1
  Controlled Voltage Source/LConn1 -- Controlled PWM Voltage/LConn1
  Simulink-PS Converter/RConn1 -- Controlled Voltage Source/RConn1
  Ideal Torque Sensor/RConn2 -- Torque/RConn1
  DC Motor/LConn2 -- Gear Box/LConn1
  Gear Box/RConn1 -- Ideal Torque Sensor/LConn1
  Simulink-PS Converter1/RConn1 -- Controlled Voltage Source1/RConn1
  Controlled Voltage Source1/LConn1 -- H-Bridge/LConn3

== system Modelo_R2023b/Nexus/Nexus Robot/Wheel ω4 Back Right/DC_Motor Pololu 37DX70L 70:1 - 64 CPR/Mechanics ==
  Axis : sm_lib/Body Elements/File Solid  ExtGeomFileName=c_MG37D_Eje.stp  UnitType=FromFile  ExtGeomFileUnits=m  StepReaderType=HEX  ExportConvexHullGeometry=off  InertiaType=CalculateFromGeometry  Mass=1  MassUnits=kg  CenterOfMass=[0 0 0]  CenterOfMassUnits=m  MomentsOfInertia=[1 1 1]  MomentsOfInertiaUnits=kg*m^2  ProductsOfInertia=[0 0 0]  ProductsOfInertiaUnits=kg*m^2  BasedOnType=Density  Density=7850  DensityUnits=kg/m^3  DoExposeReferenceFrame=on  SerializedFrames=<Frames><Frame><Id>Frame1</Id><Value><Name>F1</Name><Origin><Source>GeometricFeature</Source><FeatureName>circular curve 6</FeatureName></Origin><PrimaryAxis><DefinedDirection>+Z</DefinedDirection><Source>ReferenceFrame</Source><SourceDirection>+Z</SourceDirection><FeatureName></FeatureName></PrimaryAxis><SecondaryAxis><DefinedDirection>+X</DefinedDirection><Source>ReferenceFrame</Source><SourceDirection>+X</SourceDirection><FeatureName></FeatureName></SecondaryAxis></Value></Frame></Frames>  GraphicType=FromGeometry  MarkerShape=Sphere  MarkerSize=10  GraphicVisPropType=SimpleVisualProperties  GraphicDiffuseColor=[0.8 0.8 0.8]  GraphicSpecularColor=[0.5 0.5 0.5 1.0]  GraphicAmbientColor=[0.15 0.15 0.15 1.0]  GraphicEmissiveColor=[0.0 0.0 0.0 1.0]  GraphicShininess=75  GraphicOpacity=1.0
  PS Gain : fl_lib/Physical Signals/Functions/PS Gain  gain=DC_Motor_TG
  Revolute Joint : sm_lib/Joints/Revolute Joint  JointMode=Normal  SenseConstraintForce=off  SenseConstraintForceX=off  SenseConstraintForceY=off  SenseConstraintForceZ=off  SenseConstraintTorque=off  SenseConstraintTorqueX=off  SenseConstraintTorqueY=off  SenseConstraintTorqueZ=off  SenseTotalForce=off  SenseTotalForceX=off  SenseTotalForceY=off  SenseTotalForceZ=off  SenseTotalTorque=off  SenseTotalTorqueX=off  SenseTotalTorqueY=off  SenseTotalTorqueZ=off  CompositeWrenchDir=FollowerOnBase  CompositeWrenchFrame=BaseFrame  EquilibriumPosition=0  EquilibriumPositionUnits=deg  SpringStiffness=0  SpringStiffnessUnits=N*m/deg  DampingCoefficient=DC_Joint_J  DampingCoefficientUnits=N*m/(rad/s)  TorqueActuationMode=InputTorque  MotionActuationMode=ComputedMotion  SensePosition=on  SenseVelocity=on  SenseAcceleration=off  SenseTorqueForce=off  SenseLowerLimitTorqueForce=off  SenseUpperLimitTorqueForce=off  LowerLimitSpecify=off  LowerLimitBound=-90  LowerLimitBoundUnits=deg  LowerLimitStiffness=1e4  LowerLimitStiffnessUnits=N*m/deg  LowerLimitDamping=10  LowerLimitDampingUnits=N*m/(deg/s)  LowerLimitTransitionRegionWidth=0.1  LowerLimitTransitionRegionWidthUnits=deg  UpperLimitSpecify=off  UpperLimitBound=90  UpperLimitBoundUnits=deg  UpperLimitStiffness=1e4  UpperLimitStiffnessUnits=N*m/deg  UpperLimitDamping=10  UpperLimitDampingUnits=N*m/(deg/s)  UpperLimitTransitionRegionWidth=0.1  UpperLimitTransitionRegionWidthUnits=deg  PositionTargetSpecify=off  PositionTargetPriority=High  PositionTargetValue=0  PositionTargetValueUnits=deg  VelocityTargetSpecify=off  VelocityTargetPriority=High  VelocityTargetValue=0  VelocityTargetValueUnits=deg/s
  FW : PMIOPort  Side=Left
  τ : PMIOPort  Port=2  Side=Left
  Wheel : PMIOPort  Port=3  Side=Right
  θ : PMIOPort  Port=4  Side=Right
  ω : PMIOPort  Port=5  Side=Right
  connections:
  Revolute Joint/RConn2 -- θ/RConn1
  FW/RConn1 -- Revolute Joint/LConn1
  Axis/RConn1 -- Revolute Joint/RConn1
  PS Gain/LConn1 -- τ/RConn1
  Revolute Joint/RConn3 -- ω/RConn1
  Revolute Joint/LConn2 -- PS Gain/RConn1
  Wheel/RConn1 -- Axis/LConn1

== matlab function Modelo_R2023b/Nexus/Nexus Robot/Wheel ω2 Front Right/DC_Motor Pololu 37DX70L 70:1 - 64 CPR/Electrical/Deadzone ==
  data: u_min input; u input; y output
function y = fcn(u_min,u)
if u < u_min
    u = 0;
end
y = u;

== matlab function Modelo_R2023b/Nexus/Nexus Robot/Wheel ω3 Back Left/DC_Motor Pololu 37DX70L 70:1 - 64 CPR/Electrical/Deadzone ==
  data: u_min input; u input; y output
function y = fcn(u_min,u)
if u < u_min
    u = 0;
end
y = u;

== matlab function Modelo_R2023b/Nexus/Nexus Robot/Wheel ω4 Back Right/DC_Motor Pololu 37DX70L 70:1 - 64 CPR/Electrical/Deadzone ==
  data: u_min input; u input; y output
function y = fcn(u_min,u)
if u < u_min
    u = 0;
end
y = u;

== matlab function Modelo_R2023b/Nexus/Nexus Robot/Wheel ω1 Front Left/DC_Motor Pololu 37DX70L 70:1 - 64 CPR/Electrical/Deadzone ==
  data: u_min input; u input; y output
function y = fcn(u_min,u)
if u < u_min
    u = 0;
end
y = u;
